simulink model "Spine2sim"  (R2015a)
settings: Solver=ode45  StartTime=0.0  StopTime=tstep  RelTol=1e-10  AbsTol=1e-10
values from neighbouring files (symbols this model uses):
  d = 0.0257    [SimulinkTests.m]
  I = (0.5^2*0.33)*3    (= 0.2475)    [MAINode.m]    (also in SimulinkTests.m = 10000)
  k = 1500    [MAINode.m]    (also in SimulinkTests.m)
  ks = 1500    [MAINode.m]    (also in SimulinkTests.m)
  l = 1    [MAINode.m]    (also in SimulinkTests.m)
  m = 3    [MAINode.m]    (also in SimulinkTests.m)
  theta0 = 0    [SimulinkTests.m]
  x2 = [0 2]    [SimulinkTests.m]
libraries: vrlib x5, aerolibutil x5
settings Model: Creator=Zeerek  LastModifiedBy=Zeerek
settings DataIOCC: LimitDataPoints=off

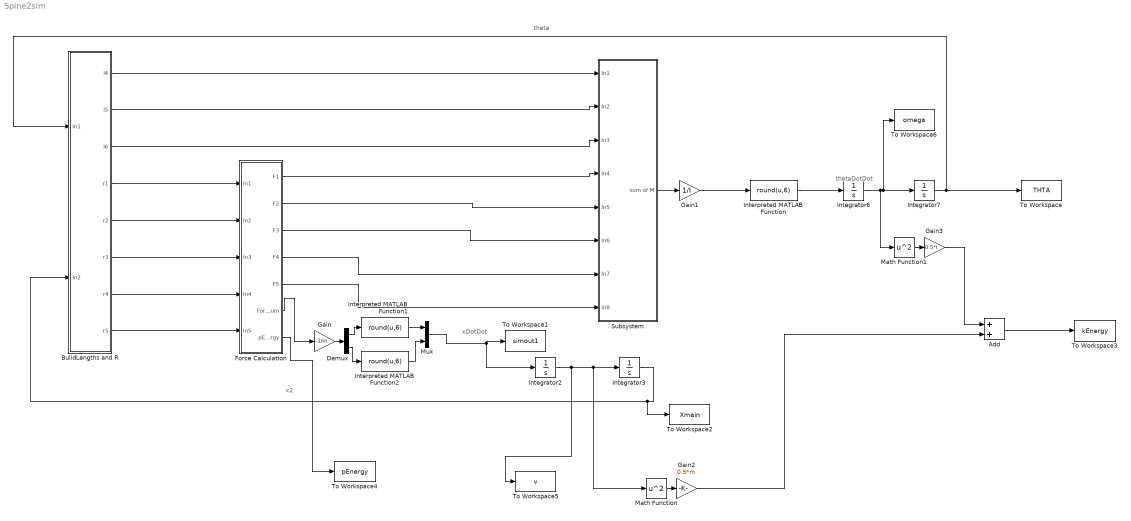
== system Spine2sim ==
  note: theta
  note: x2
  note: xDotDot
  note: thetaDotDot
  Add : Sum
  BulidLengths and R : Subsystem
  Demux : Demux  Outputs=2
  Force Calculation : Subsystem
  Gain : Gain  Gain=-1/m
  Gain1 : Gain  Gain=1/I
  Gain2 : Gain  Gain=0.5*m
  Gain3 : Gain  Gain=0.5*I
  Integrator2 : Integrator  InitialCondition=[0 0]
  Integrator3 : Integrator  InitialCondition=[x2(1) x2(2)]
  Integrator6 : Integrator
  Integrator7 : Integrator  InitialCondition=theta0
  Interpreted MATLAB Function : MATLABFcn  MATLABFcn=round(u,6)  Output1D=off
  Interpreted MATLAB Function1 : MATLABFcn  MATLABFcn=round(u,6)  Output1D=off
  Interpreted MATLAB Function2 : MATLABFcn  MATLABFcn=round(u,6)  Output1D=off
  Math Function : Math  Operator=square  SaturateOnIntegerOverflow=on
  Math Function1 : Math  Operator=square  SaturateOnIntegerOverflow=on
  Mux : Mux  Inputs=2
  Subsystem : Subsystem
  To Workspace : ToWorkspace  VariableName=THTA  SaveFormat=Timeseries  SampleTime=-1
  To Workspace1 : ToWorkspace  VariableName=simout1  SaveFormat=Timeseries  SampleTime=-1
  To Workspace2 : ToWorkspace  VariableName=Xmain  SaveFormat=Timeseries  SampleTime=-1
  To Workspace3 : ToWorkspace  VariableName=kEnergy  SaveFormat=Timeseries  SampleTime=-1
  To Workspace4 : ToWorkspace  VariableName=pEnergy  SaveFormat=Timeseries  SampleTime=-1
  To Workspace5 : ToWorkspace  VariableName=v  SaveFormat=Timeseries  SampleTime=-1
  To Workspace6 : ToWorkspace  VariableName=omega  SaveFormat=Timeseries  SampleTime=-1
  wires:
  BulidLengths and R/4(r1) -> Force Calculation/1(In1)
  BulidLengths and R/5(r2) -> Force Calculation/2(In2)
  BulidLengths and R/6(r3) -> Force Calculation/3(In3)
  BulidLengths and R/7(r4) -> Force Calculation/4(In4)
  BulidLengths and R/8(r5) -> Force Calculation/5(In5)
  Force Calculation/6(ForceSum) -> Gain/1
  BulidLengths and R/1("l4 ") -> Subsystem/1(In1)
  BulidLengths and R/2(l5) -> Subsystem/2(In2)
  BulidLengths and R/3(l6) -> Subsystem/3(In3)
  Force Calculation/1(F1) -> Subsystem/4(In4)
  Force Calculation/2(F2) -> Subsystem/5(In5)
  Force Calculation/3(F3) -> Subsystem/6(In6)
  Force Calculation/4(F4) -> Subsystem/7(In7)
  Force Calculation/5(F5) -> Subsystem/8(In8)
  Gain1/1 -> Interpreted MATLAB Function/1
  Integrator2/1 -> To Workspace5/1, Math Function/1, Integrator3/1
  Integrator3/1 -> To Workspace2/1, BulidLengths and R/2(In2)
  Integrator7/1 -> BulidLengths and R/1(In1), To Workspace/1
  Math Function/1 -> Gain2/1
  Math Function1/1 -> Gain3/1
  Integrator6/1 -> Math Function1/1, Integrator7/1, To Workspace6/1
  Gain3/1 -> Add/1
  Gain2/1 -> Add/2
  Force Calculation/7(pEnergy) -> To Workspace4/1
  Add/1 -> To Workspace3/1
  Gain/1 -> Demux/1
  Subsystem/1(sum of M) -> Gain1/1
  Interpreted MATLAB Function/1 -> Integrator6/1
  Mux/1 -> To Workspace1/1, Integrator2/1
  Demux/1 -> Interpreted MATLAB Function1/1
  Demux/2 -> Interpreted MATLAB Function2/1
  Interpreted MATLAB Function1/1 -> Mux/1
  Interpreted MATLAB Function2/1 -> Mux/2

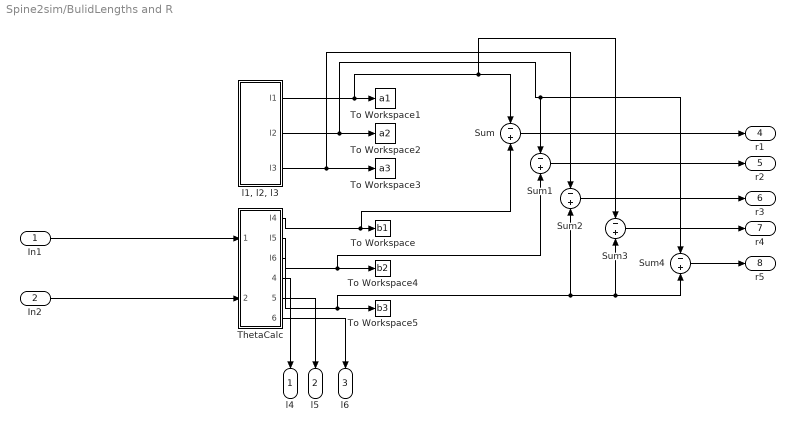
== system Spine2sim/BulidLengths and R ==
  In1 : Inport
  In2 : Inport  Port=2
  Sum{,1..4} (5 alike) : Sum  Inputs=-+
  ThetaCalc : Subsystem
  To Workspace : ToWorkspace  VariableName=b1  SaveFormat=Timeseries  SampleTime=-1
  To Workspace1 : ToWorkspace  VariableName=a1  SaveFormat=Timeseries  SampleTime=-1
  To Workspace2 : ToWorkspace  VariableName=a2  SaveFormat=Timeseries  SampleTime=-1
  To Workspace3 : ToWorkspace  VariableName=a3  SaveFormat=Timeseries  SampleTime=-1
  To Workspace4 : ToWorkspace  VariableName=b2  SaveFormat=Timeseries  SampleTime=-1
  To Workspace5 : ToWorkspace  VariableName=b3  SaveFormat=Timeseries  SampleTime=-1
  "l1, l2, l3" : Subsystem
  "l4 " : Outport
  l5 : Outport  Port=2
  l6 : Outport  Port=3
  r1 : Outport  Port=4
  r2 : Outport  Port=5
  r3 : Outport  Port=6
  r4 : Outport  Port=7
  r5 : Outport  Port=8
  wires:
  "l1, l2, l3"/1(l1) -> Sum3/1, Sum/1, To Workspace1/1
  ThetaCalc/3(l6) -> Sum2/2, Sum3/2, Sum4/2, To Workspace5/1
  ThetaCalc/2(l5) -> To Workspace4/1, Sum1/2
  In2/1 -> ThetaCalc/2(In2)
  "l1, l2, l3"/2(l2) -> To Workspace2/1, Sum4/1, Sum1/1
  "l1, l2, l3"/3(l3) -> To Workspace3/1, Sum2/1
  In1/1 -> ThetaCalc/1(In1)
  Sum4/1 -> r5/1
  Sum3/1 -> r4/1
  Sum/1 -> r1/1
  Sum1/1 -> r2/1
  Sum2/1 -> r3/1
  ThetaCalc/1(l4) -> Sum/2, To Workspace/1
  ThetaCalc/4(Out1) -> "l4 "/1
  ThetaCalc/5(Out2) -> l5/1
  ThetaCalc/6(Out3) -> l6/1

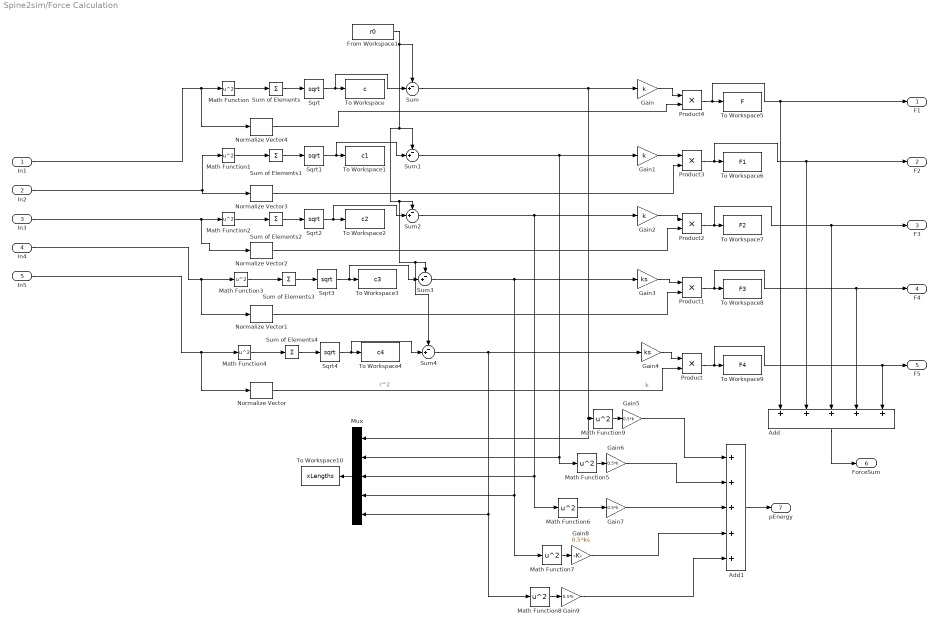
== system Spine2sim/Force Calculation ==
  note: k
  note: r^2
  In1 : Inport
  In2 : Inport  Port=2
  In3 : Inport  Port=3
  In4 : Inport  Port=4
  In5 : Inport  Port=5
  Add : Sum  Inputs=+++++
  Add1 : Sum  Inputs=+++++
  From Workspace1 : FromWorkspace  VariableName=r0  SampleTime=0
  Gain : Gain  Gain=k
  Gain1 : Gain  Gain=k
  Gain2 : Gain  Gain=k
  Gain3 : Gain  Gain=ks
  Gain4 : Gain  Gain=ks
  Gain{5..7,9} (4 alike) : Gain  Gain=0.5*k
  Gain8 : Gain  Gain=0.5*ks
  Math Function{,1..9} (10 alike) : Math  Operator=square  SaturateOnIntegerOverflow=on
  Mux : Mux  Inputs=5
  Normalize Vector{,1..4} (5 alike) : vrlib/Utilities/Normalize Vector  maxzero=0
  Product{,1..4} (5 alike) : Product
  Sqrt{,1..4} (5 alike) : Sqrt  SaturateOnIntegerOverflow=on
  Sum{,1..4} (5 alike) : Sum  Inputs=-+|
  Sum of Elements{,1..4} (5 alike) : Sum  Inputs=+
  To Workspace : ToWorkspace  VariableName=c  SaveFormat=Timeseries  SampleTime=-1
  To Workspace1 : ToWorkspace  VariableName=c1  SaveFormat=Timeseries  SampleTime=-1
  To Workspace10 : ToWorkspace  VariableName=xLengths  SaveFormat=Timeseries  SampleTime=-1
  To Workspace2 : ToWorkspace  VariableName=c2  SaveFormat=Timeseries  SampleTime=-1
  To Workspace3 : ToWorkspace  VariableName=c3  SaveFormat=Timeseries  SampleTime=-1
  To Workspace4 : ToWorkspace  VariableName=c4  SaveFormat=Timeseries  SampleTime=-1
  To Workspace5 : ToWorkspace  VariableName=F  SaveFormat=Timeseries  SampleTime=-1
  To Workspace6 : ToWorkspace  VariableName=F1  SaveFormat=Timeseries  SampleTime=-1
  To Workspace7 : ToWorkspace  VariableName=F2  SaveFormat=Timeseries  SampleTime=-1
  To Workspace8 : ToWorkspace  VariableName=F3  SaveFormat=Timeseries  SampleTime=-1
  To Workspace9 : ToWorkspace  VariableName=F4  SaveFormat=Timeseries  SampleTime=-1
  F1 : Outport
  F2 : Outport  Port=2
  F3 : Outport  Port=3
  F4 : Outport  Port=4
  F5 : Outport  Port=5
  ForceSum : Outport  Port=6
  pEnergy : Outport  Port=7
  wires:
  Sum of Elements2/1 -> Sqrt2/1
  Sqrt/1 -> Sum/2, To Workspace/1
  Math Function4/1 -> Sum of Elements4/1
  Sqrt1/1 -> Sum1/2, To Workspace1/1
  Sqrt3/1 -> Sum3/2, To Workspace3/1
  Math Function1/1 -> Sum of Elements1/1
  Sum of Elements4/1 -> Sqrt4/1
  In5/1 -> Normalize Vector/1, Math Function4/1
  Math Function/1 -> Sum of Elements/1
  Math Function2/1 -> Sum of Elements2/1
  Math Function3/1 -> Sum of Elements3/1
  Sum of Elements/1 -> Sqrt/1
  Sum of Elements1/1 -> Sqrt1/1
  Sum of Elements3/1 -> Sqrt3/1
  Sqrt4/1 -> Sum4/2, To Workspace4/1
  In1/1 -> Normalize Vector4/1, Math Function/1
  Normalize Vector4/1 -> Product4/2
  Gain3/1 -> Product1/1
  In4/1 -> Normalize Vector1/1, Math Function3/1
  Normalize Vector/1 -> Product/2
  From Workspace1/1 -> Sum/1, Sum4/1, Sum3/1, Sum2/1, Sum1/1
  In2/1 -> Normalize Vector3/1, Math Function1/1
  Normalize Vector2/1 -> Product2/2
  Sqrt2/1 -> Sum2/2, To Workspace2/1
  Product1/1 -> Add/4, F4/1, To Workspace8/1
  Gain1/1 -> Product3/1
  Sum2/1 -> Math Function6/1, Mux/3, Gain2/1
  Gain/1 -> Product4/1
  Product3/1 -> Add/2, F2/1, To Workspace6/1
  In3/1 -> Normalize Vector2/1, Math Function2/1
  Sum/1 -> Mux/1, Math Function9/1, Gain/1
  Gain2/1 -> Product2/1
  Normalize Vector1/1 -> Product1/2
  Sum1/1 -> Mux/2, Math Function5/1, Gain1/1
  Gain4/1 -> Product/1
  Product/1 -> Add/5, F5/1, To Workspace9/1
  Normalize Vector3/1 -> Product3/2
  Product4/1 -> Add/1, F1/1, To Workspace5/1
  Product2/1 -> F3/1, Add/3, To Workspace7/1
  Add/1 -> ForceSum/1
  Math Function9/1 -> Gain5/1
  Math Function5/1 -> Gain6/1
  Math Function6/1 -> Gain7/1
  Math Function7/1 -> Gain8/1
  Math Function8/1 -> Gain9/1
  Gain5/1 -> Add1/1
  Gain6/1 -> Add1/2
  Gain7/1 -> Add1/3
  Gain8/1 -> Add1/4
  Gain9/1 -> Add1/5
  Add1/1 -> pEnergy/1
  Sum3/1 -> Mux/4, Math Function7/1, Gain3/1
  Sum4/1 -> Math Function8/1, Mux/5, Gain4/1
  Mux/1 -> To Workspace10/1

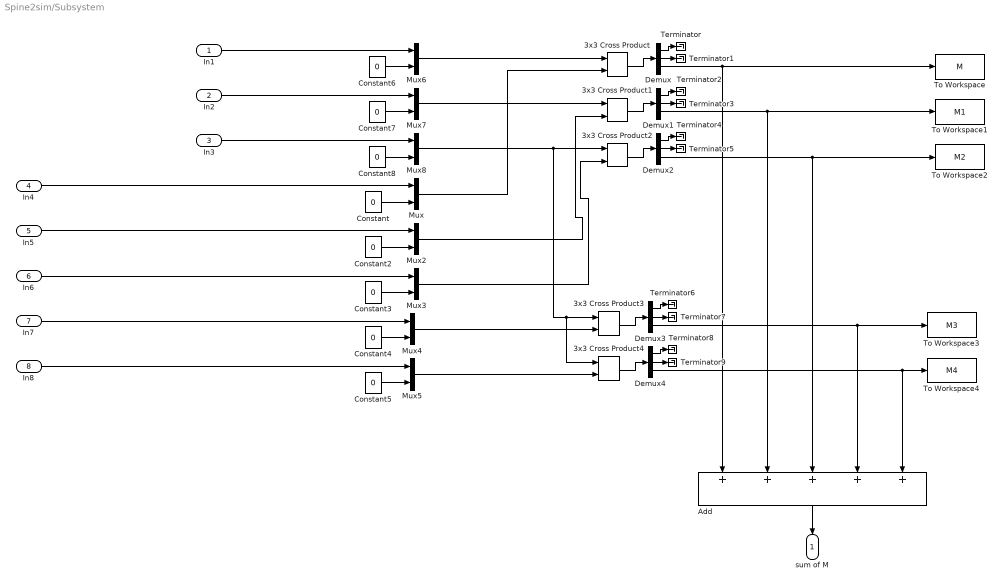
== system Spine2sim/Subsystem ==
  In1 : Inport
  In2 : Inport  Port=2
  In3 : Inport  Port=3
  In4 : Inport  Port=4
  In5 : Inport  Port=5
  In6 : Inport  Port=6
  In7 : Inport  Port=7
  In8 : Inport  Port=8
  3x3 Cross Product{,1..4} (5 alike) : aerolibutil/3x3 Cross Product
  Add : Sum  Inputs=+++++
  Constant{,2..8} (8 alike) : Constant  Value=0
  Demux{,1..4} (5 alike) : Demux  Outputs=3
  Mux{,2..8} (8 alike) : Mux  Inputs=2
  Terminator{,1..9} (10 alike) : Terminator
  To Workspace : ToWorkspace  VariableName=M  SaveFormat=Timeseries  SampleTime=-1
  To Workspace1 : ToWorkspace  VariableName=M1  SaveFormat=Timeseries  SampleTime=-1
  To Workspace2 : ToWorkspace  VariableName=M2  SaveFormat=Timeseries  SampleTime=-1
  To Workspace3 : ToWorkspace  VariableName=M3  SaveFormat=Timeseries  SampleTime=-1
  To Workspace4 : ToWorkspace  VariableName=M4  SaveFormat=Timeseries  SampleTime=-1
  sum of M : Outport
  wires:
  Mux7/1 -> 3x3 Cross Product1/1
  In7/1 -> Mux4/1
  Constant/1 -> Mux/2
  Constant4/1 -> Mux4/2
  Constant3/1 -> Mux3/2
  In6/1 -> Mux3/1
  Mux/1 -> 3x3 Cross Product/2
  Demux/1 -> Terminator/1
  3x3 Cross Product1/1 -> Demux1/1
  Demux1/3 -> Add/2, To Workspace1/1
  Mux6/1 -> 3x3 Cross Product/1
  Demux2/3 -> Add/3, To Workspace2/1
  3x3 Cross Product2/1 -> Demux2/1
  Constant8/1 -> Mux8/2
  In3/1 -> Mux8/1
  In1/1 -> Mux6/1
  Constant6/1 -> Mux6/2
  Constant7/1 -> Mux7/2
  In2/1 -> Mux7/1
  In4/1 -> Mux/1
  Demux3/1 -> Terminator6/1
  Demux3/2 -> Terminator7/1
  Mux2/1 -> 3x3 Cross Product1/2
  In8/1 -> Mux5/1
  Constant5/1 -> Mux5/2
  In5/1 -> Mux2/1
  Constant2/1 -> Mux2/2
  Mux3/1 -> 3x3 Cross Product2/2
  3x3 Cross Product4/1 -> Demux4/1
  3x3 Cross Product/1 -> Demux/1
  Demux3/3 -> Add/4, To Workspace3/1
  3x3 Cross Product3/1 -> Demux3/1
  Mux8/1 -> 3x3 Cross Product2/1, 3x3 Cross Product4/1, 3x3 Cross Product3/1
  Mux4/1 -> 3x3 Cross Product3/2
  Demux/3 -> Add/1, To Workspace/1
  Demux/2 -> Terminator1/1
  Demux4/1 -> Terminator8/1
  Demux4/2 -> Terminator9/1
  Demux1/2 -> Terminator3/1
  Demux2/2 -> Terminator5/1
  Demux2/1 -> Terminator4/1
  Demux1/1 -> Terminator2/1
  Mux5/1 -> 3x3 Cross Product4/2
  Demux4/3 -> Add/5, To Workspace4/1
  Add/1 -> sum of M/1

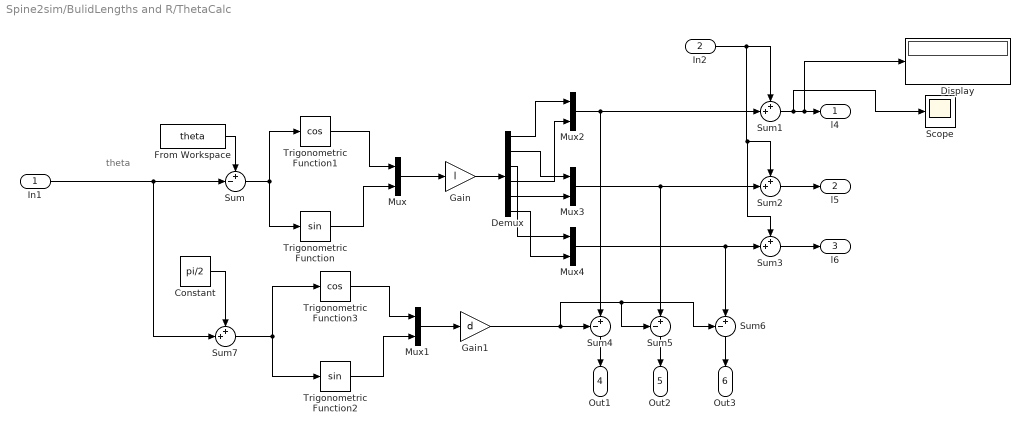
== system Spine2sim/BulidLengths and R/ThetaCalc ==
  note: theta
  In1 : Inport
  In2 : Inport  Port=2
  Constant : Constant  Value=pi/2
  Demux : Demux  Outputs=6
  Display : Display
  From Workspace : FromWorkspace  VariableName=theta  SampleTime=0
  Gain : Gain  Gain=l
  Gain1 : Gain  Gain=d
  Mux{,1..4} (5 alike) : Mux  Inputs=2
  Scope : Scope
  Sum : Sum  Inputs=+-|
  Sum{1..3,7} (4 alike) : Sum  Inputs=++|
  Sum4 : Sum  Inputs=-+|
  Sum5 : Sum  Inputs=-+|
  Sum6 : Sum  Inputs=-+|
  Trigonometric Function : Trigonometry
  Trigonometric Function1 : Trigonometry  Operator=cos
  Trigonometric Function2 : Trigonometry
  Trigonometric Function3 : Trigonometry  Operator=cos
  l4 : Outport
  l5 : Outport  Port=2
  l6 : Outport  Port=3
  Out1 : Outport  Port=4
  Out2 : Outport  Port=5
  Out3 : Outport  Port=6
  wires:
  Gain/1 -> Demux/1
  Sum/1 -> Trigonometric Function1/1, Trigonometric Function/1
  Demux/2 -> Mux3/1
  Demux/5 -> Mux3/2
  Demux/4 -> Mux2/2
  Demux/6 -> Mux4/2
  Demux/1 -> Mux2/1
  Demux/3 -> Mux4/1
  Trigonometric Function/1 -> Mux/2
  Trigonometric Function1/1 -> Mux/1
  Mux3/1 -> Sum5/2, Sum2/2
  Mux2/1 -> Sum4/2, Sum1/2
  In2/1 -> Sum1/1, Sum3/1, Sum2/1
  Sum1/1 -> Scope/1, Display/1, l4/1
  Mux4/1 -> Sum6/2, Sum3/2
  Sum2/1 -> l5/1
  Sum3/1 -> l6/1
  Mux/1 -> Gain/1
  Sum4/1 -> Out1/1
  Sum5/1 -> Out2/1
  Sum6/1 -> Out3/1
  Gain1/1 -> Sum6/1, Sum5/1, Sum4/1
  From Workspace/1 -> Sum/1
  Trigonometric Function2/1 -> Mux1/2
  Trigonometric Function3/1 -> Mux1/1
  Mux1/1 -> Gain1/1
  In1/1 -> Sum7/2, Sum/2
  Sum7/1 -> Trigonometric Function3/1, Trigonometric Function2/1
  Constant/1 -> Sum7/1

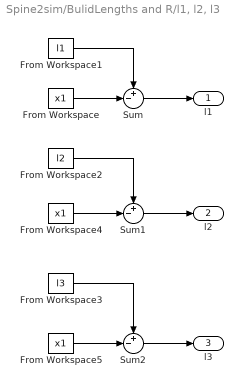
== system Spine2sim/BulidLengths and R/l1, l2, l3 ==
  From Workspace : FromWorkspace  VariableName=x1  SampleTime=0
  From Workspace1 : FromWorkspace  VariableName=l1  SampleTime=0
  From Workspace2 : FromWorkspace  VariableName=l2  SampleTime=0
  From Workspace3 : FromWorkspace  VariableName=l3  SampleTime=0
  From Workspace4 : FromWorkspace  VariableName=x1  SampleTime=0
  From Workspace5 : FromWorkspace  VariableName=x1  SampleTime=0
  Sum : Sum  Inputs=+-|
  Sum1 : Sum  Inputs=+-|
  Sum2 : Sum  Inputs=+-|
  l1 : Outport
  l2 : Outport  Port=2
  l3 : Outport  Port=3
  wires:
  From Workspace4/1 -> Sum1/2
  From Workspace1/1 -> Sum/1
  From Workspace2/1 -> Sum1/1
  From Workspace/1 -> Sum/2
  Sum/1 -> l1/1
  Sum1/1 -> l2/1
  Sum2/1 -> l3/1
  From Workspace3/1 -> Sum2/1
  From Workspace5/1 -> Sum2/2
